simulink model "Simulation"  (R2015b)
settings: Solver=VariableStepAuto  StartTime=0.0  StopTime=100  RelTol=1e-3
settings Model: Creator=TOSHIBA  LastModifiedBy=TOSHIBA

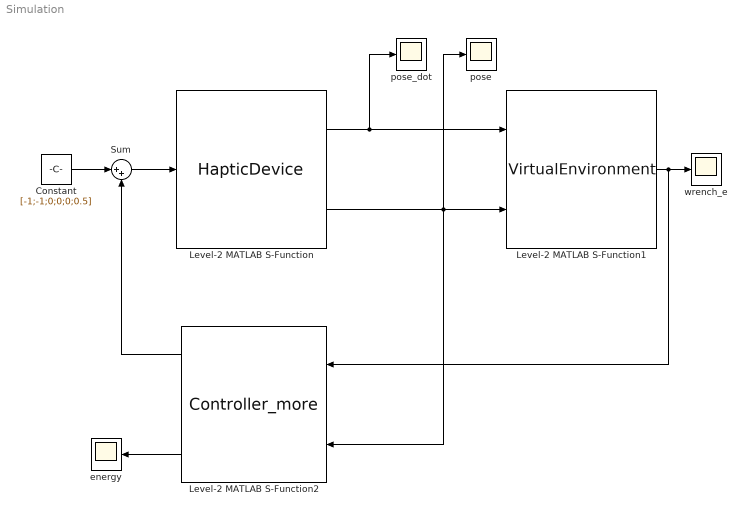
== system Simulation ==
  Constant : Constant  Value=[-1;-1;0;0;0;0.5]
  Level-2 MATLAB S-Function : M-S-Function  FunctionName=HapticDevice  Parameters=miDevice, bDevice, pose_dot0, pose0, dof
  Level-2 MATLAB S-Function1 : M-S-Function  FunctionName=VirtualEnvironment  Parameters=kWall, bWall, nWall, pWall, vertices, dof, tsampling
  Level-2 MATLAB S-Function2 : M-S-Function  FunctionName=Controller_more  Parameters=bDevice, pose0, dof, tsampling
  Sum : Sum  Inputs=|++
  energy : Scope
  pose : Scope
  pose_dot : Scope
  wrench_e : Scope
  wires:
  Level-2 MATLAB S-Function/1 -> pose_dot/1, Level-2 MATLAB S-Function1/1
  Level-2 MATLAB S-Function/2 -> Level-2 MATLAB S-Function2/2, Level-2 MATLAB S-Function1/2, pose/1
  Sum/1 -> Level-2 MATLAB S-Function/1
  Constant/1 -> Sum/1
  Level-2 MATLAB S-Function1/1 -> Level-2 MATLAB S-Function2/1, wrench_e/1
  Level-2 MATLAB S-Function2/3 -> energy/1
  Level-2 MATLAB S-Function2/1 -> Sum/2
